simulink model "complementrary_sensitivity"  (R2021a)
settings: Solver=FixedStepAuto  StartTime=0.0  StopTime=StopTime  FixedStep=Ts  RelTol=1e-3
values from neighbouring files (symbols this model uses):
  CFB = ss(CFB)    [NAPAS_closed_loop.m]    (also in NAPAS_closed_loop_T_and_S.m)
  Plant_ct = ss(Ap,Bp,Cp,zeros(6,6))    [NAPAS_closed_loop.m]    (also in NAPAS_closed_loop_T_and_S.m)
  Ts = 1/fs    [NAPAS_closed_loop.m]    (also in NAPAS_closed_loop_T_and_S.m; test_2_2_system.m; test_6_outputs_8_inputs_identification.m; test_multisine.m)
settings Model: Creator=20155774  LastModifiedBy=42447
settings SolverCC: AlgebraicLoopSolver=TrustRegion
settings DebuggingCC: SFMachineParentedDataDiag=warning

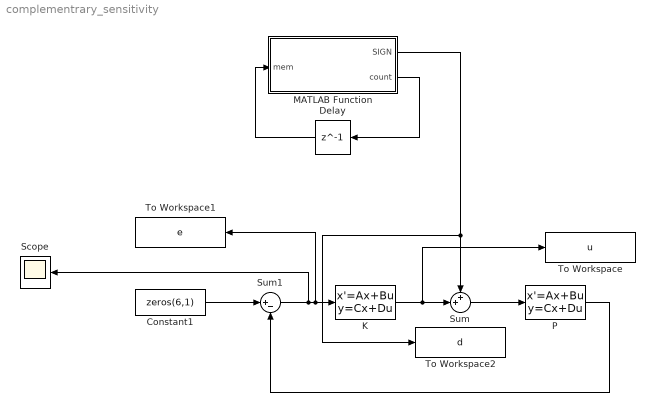
== system complementrary_sensitivity ==
  Constant1 : Constant  Value=zeros(6,1)
  Delay : Delay  DelayLength=1  InitialCondition=1  SampleTime=Ts
  K : StateSpace  A=CFB.A  B=CFB.B  C=CFB.C  D=CFB.D  InitialCondition=0
  MATLAB Function : MATLAB Function  TreatAsAtomicUnit=on
  P : StateSpace  A=Plant_ct.A  B=Plant_ct.B  C=Plant_ct.C  D=Plant_ct.D  InitialCondition=0
  Scope : Scope
  Sum : Sum  Inputs=++|
  Sum1 : Sum  Inputs=|+-
  To Workspace : ToWorkspace  VariableName=u  SaveFormat=Structure With Time  SampleTime=-1
  To Workspace1 : ToWorkspace  VariableName=e  SaveFormat=Structure With Time  SampleTime=-1
  To Workspace2 : ToWorkspace  VariableName=d  SaveFormat=Structure With Time  SampleTime=-1
  wires:
  K/1 -> To Workspace/1, Sum/2
  Sum/1 -> P/1
  P/1 -> Sum1/2
  Sum1/1 -> K/1, To Workspace1/1, Scope/1
  MATLAB Function/2(count) -> Delay/1
  Delay/1 -> MATLAB Function/1(mem)
  MATLAB Function/1(SIGN) -> To Workspace2/1, Sum/1
  Constant1/1 -> Sum1/1

== matlab function complementrary_sensitivity/MATLAB Function ==
  data: SIGN output; mem input; count output; EXCSIG parameter
function [SIGN,count] = fcn(mem, EXCSIG)

SIGN    =   EXCSIG(:,mem);
count   =   mem + 1;
